simulink model "MicrogridControl"  (R2025b)
settings: Solver=VariableStepAuto  StartTime=0.0  StopTime=8  FixedStep=Ts  RelTol=1e-3
PreLoadFcn:
  | NormalOperation;
  | MicrogridControlParam;
undefined symbols (not defined in the file): base, bessModeInitial, bessSystem, bessVoltage, breakerStatus, DiscIntNeverNeededParam, ee_sli_rtmsupport, event, gcbh, generator, gflInverter, gfmInverter, Inertia, lineInductance, lineResistance, machine, plannedIsland, pmsm, powerLimit, powerQuality, PV, PVInverter, ref, resync, solar, solarInsolationChange, systemFrequency, Ts, windController, windSystem, windTurbine
libraries: nesl_utility x234, ee_lib x174, fl_lib x143, eeGeneralControl x137, simulink x78, eeTransforms x47, slpidlib x23, nesl_utility_internal x12, eePwmGenerator x9, eeSinusoidalMeasurementV2 x9, custom_lib x7, batteryecm_lib x6
(part 4 of 25)

== system MicrogridControl/Wind Farm ==
  Constant : Constant  Value=10
  Constant1 : Constant  Value=0
  Constant2 : Constant  Value=12
  Transformer : Subsystem  Variant=on  VariantControlMode=label  LabelModeActiveChoice=Detailed  mask{fidelity=Detailed}
      mask prompts: fidelity "Modeling Option"
      mask TypeOptions fidelity: Detailed | Simplified
      mask Callback fidelity:
      | choice = get_param(gcb,'fidelity');
      | switch choice
      |     case 'Detailed'
      |         set_param(gcb, 'LabelModeActiveChoice', 'Detailed');
      |     case 'Simplified'
      |          set_param(gcb, 'LabelModeActiveChoice', 'Simplified');
      |     otherwise
      |         disp('Choose proper variant');
      | end
  Transformer1 : Subsystem  Variant=on  VariantControlMode=label  LabelModeActiveChoice=Detailed  mask{fidelity=Detailed}
      mask prompts: fidelity "Modeling Option"
      mask TypeOptions fidelity: Detailed | Simplified
      mask Callback fidelity:
      | choice = get_param(gcb,'fidelity');
      | switch choice
      |     case 'Detailed'
      |         set_param(gcb, 'LabelModeActiveChoice', 'Detailed');
      |     case 'Simplified'
      |          set_param(gcb, 'LabelModeActiveChoice', 'Simplified');
      |     otherwise
      |         disp('Choose proper variant');
      | end
  Wind Plant Integrated : Subsystem  Variant=on  VariantControlMode=label  LabelModeActiveChoice=Detailed  mask(Wind){fidelity=Detailed, plantRating=windSystem.plantRating, Vac=windSystem.Vac, frequency=windSystem.frequency, iMaxPU=windSystem.iMaxPU, efficiency=windSystem.converterEfficiency, baseVoltageDC=windSystem.Vdc, airDensity=windTurbine.airDensity, turbineRadius=windTurbine.turbineRadius, pitch=windTurbine.pitch, TSR=windTurbine.TSR, cp=windTurbine.cp, wt=windTurbine.wThreshold, rt=windTurbine.wThreshold, p=pmsm.polePairs, psim=pmsm.fluxLinkage, Rs=pmsm.Rs, Ld=pmsm.Ld, Lq=pmsm.Lq, capacitance=windSystem.capacitance, filterInductance=windSystem.filterInductance, filterResistance=windSystem.filterResistance, converterFidelity=Average, fSw=20}
      mask prompts: fidelity "Modeling Option"; plantRating "Wind Farm Rating (kW)"; Vac "Rated AC side voltage (phase-phase RMS) (V)"; frequency "Rated electrical frequency at AC side (Hz)"; iMaxPU "Maximum converter current (pu)"; efficiency "Converter Efficiency (%)"; baseVoltageDC "Voltage on DC side (V)"; airDensity "Air density (kg/m^3)"; turbineRadius "Turbine radius (m)"; pitch "Pitch angle vector (deg)"; TSR "Tip speed ratio"; cp "Power coefficient table, Cp(beta,TSR)"; wt "Wind velocity threshold (m/s)"; rt "Rotational velocity threshold (rad/s)"; p "Number of pole pairs"; psim "PMSM flux linkage (Wb)"; Rs "Stator resistance (Ohm)"; Ld "Stator d-axis inductance (H)"; Lq "Stator q-axis inductance (H)"; capacitance "DC bus capacitance (F)"; filterInductance "Filter inductance (H)"; filterResistance "Filter series resistance (Ohm)"; converterFidelity "Converter Fidelity"; fSw "Switching Frequency (kHz)"
      mask help: This block models a detailed Type -4 ind farm with the MPPT Controller. The wind farm comprises a permanent magnnet synhronous machine connected to the main grid via back-to-back converters. Select simplified mode for faster simulation using fixed efficiency and rated power.
      settings: CopyFcn=set_param(gcbh,'LinkStatus','none');
      mask Help: web('WindFarm.html')
      mask TypeOptions fidelity: Detailed | Simplified
      mask Callback fidelity:
      | detailedTabs = {'windDetailed','controllerDetailed','converter'};
      |     simplifiedTabs = {'windSimplified'};
      |     component.mask.fidelitySelection(detailedTabs,simplifiedTabs);
      mask TypeOptions airDensity: Detailed/Wind System/airDensity
      mask TypeOptions turbineRadius: Detailed/Wind System/turbineRadius
      mask TypeOptions pitch: Detailed/Wind System/pitch
      mask TypeOptions TSR: Detailed/Wind System/TSR
      mask TypeOptions cp: Detailed/Wind System/cp
      mask TypeOptions wt: Detailed/Wind System/wt
      mask TypeOptions rt: Detailed/Wind System/rt
      mask TypeOptions p: Detailed/Wind System/p
      mask TypeOptions psim: Detailed/Wind System/psim
      mask TypeOptions Rs: Detailed/Wind System/Rs
      mask TypeOptions Ld: Detailed/Wind System/Ld
      mask TypeOptions Lq: Detailed/Wind System/Lq
      mask TypeOptions converterFidelity: Detailed/Wind Turbine and Converters/Wind Plant/converterFidelity
      mask Callback converterFidelity:
      | converterFidelity = get_param(gcb,'converterFidelity');
      | blockPath = [gcb,'/','Detailed','/','Wind Turbine and Converters','/','Wind Plant','/','Back-to-Back Converters'];
      | % if strcmp(converterFidelity,'Average')
      | %     blockPath = [gcb,'/','Detailed','/','Wind Turbine and Converters','/','Wind Plant','/','Back-to-Back Converters'];
      | % else
      | %     blockPath = [gcb,'/','Detailed','/','Wind Turbine and Converters','/','Wind Plant','/','Back-to-Back Converters'];
      | % end
      | component.mask.converterFidelity(blockPath)
      mask TypeOptions fSw: Detailed/Wind Turbine and Converters/Wind Plant/fSw
      mask DialogControl generalDetailed Prompt: General
      mask DialogControl windDetailed Prompt: Wind Turbine
      mask DialogControl configureWindTurbine Prompt: Edit wind turbine parameters
      mask DialogControl configureWindTurbine Callback:
      | blockPath = [gcb,'/','Detailed','/','Wind Turbine and Converters','/','Wind Plant','/','Wind Turbine'];
      |     component.mask.openBlock(blockPath);
      mask DialogControl Container10 Prompt: PMSM
      mask DialogControl configurePMSM Prompt: Edit PMSM parameters
      mask DialogControl configurePMSM Callback:
      | blockPath = [gcb,'/','Detailed','/','Wind Turbine and Converters','/','Wind Plant','/','PMSG'];
      |  component.mask.openBlock(blockPath);
      mask DialogControl controllerDetailed Prompt: Controller
      mask DialogControl configureWindController Prompt: Edit Wind Controller
      mask DialogControl configureWindController Callback:
      | blockPath = [gcb,'/','Detailed','/','Wind Turbine and Converters','/','Wind Controller'];
      |     component.mask.openBlock(blockPath);
      mask DialogControl windSimplified Prompt: Wind Turbine
      mask DialogControl editWindFarm Prompt: Edit wind farm
      mask DialogControl editWindFarm Callback:
      | blockPath = [gcb,'/','Simplified','/','Wind farm'];
      | component.mask.openBlock(blockPath);
      mask DialogControl converter Prompt: Converter
      mask DialogControl editMSConverter Prompt: Edit machine side converter parameters
      mask DialogControl editMSConverter Callback:
      | blockFidelity = get_param(gcb,'fidelity');
      | converterFidelity = get_param(gcb,'converterFidelity');
      | if strcmp(converterFidelity,'Average')
      |     blockPath = [gcb,'/',blockFidelity,'/','Wind Turbine and Converters','/','Wind Plant','/','Back-to-Back Converters','/',converterFidelity,'/','Machine Side Converter'];
      | else
      |     blockPath = [gcb,'/',blockFidelity,'/','Wind Turbine and Converters','/','Wind Plant','/','Back-to-Back Converters','/',converterFidelity,'/','Machine Side Converter','/','Converter'];
      | end
      | component.mask.openBlock(blockPath);
      mask DialogControl editGSConverter Prompt: Edit grid side converter parameters
      mask DialogControl editGSConverter Callback:
      | blockFidelity = get_param(gcb,'fidelity');
      | converterFidelity = get_param(gcb,'converterFidelity');
      | if strcmp(converterFidelity,'Average')
      |     blockPath = [gcb,'/',blockFidelity,'/','Wind Turbine and Converters','/','Wind Plant','/','Back-to-Back Converters','/',converterFidelity,'/','Grid Side Converter'];
      | else
      |     blockPath = [gcb,'/',blockFidelity,'/','Wind Turbine and Converters','/','Wind Plant','/','Back-to-Back Converters','/',converterFidelity,'/','Grid Side Converter','/','Converter'];
      | end
      | component.mask.openBlock(blockPath);
      mask Display: image('wind_plant.png');
  Wind Plant Integrated1 : Subsystem  Variant=on  VariantControlMode=label  LabelModeActiveChoice=Detailed  mask(Wind){fidelity=Detailed, plantRating=windSystem.plantRating, Vac=windSystem.Vac, frequency=windSystem.frequency, iMaxPU=windSystem.iMaxPU, efficiency=windSystem.converterEfficiency, baseVoltageDC=windSystem.Vdc, airDensity=windTurbine.airDensity, turbineRadius=windTurbine.turbineRadius, pitch=windTurbine.pitch, TSR=windTurbine.TSR, cp=windTurbine.cp, wt=windTurbine.wThreshold, rt=windTurbine.wThreshold, p=pmsm.polePairs, psim=pmsm.fluxLinkage, Rs=pmsm.Rs, Ld=pmsm.Ld, Lq=pmsm.Lq, capacitance=windSystem.capacitance, filterInductance=windSystem.filterInductance, filterResistance=windSystem.filterResistance, converterFidelity=Average, fSw=20}
      mask prompts: fidelity "Modeling Option"; plantRating "Wind Farm Rating (kW)"; Vac "Rated AC side voltage (phase-phase RMS) (V)"; frequency "Rated electrical frequency at AC side (Hz)"; iMaxPU "Maximum converter current (pu)"; efficiency "Converter Efficiency (%)"; baseVoltageDC "Voltage on DC side (V)"; airDensity "Air density (kg/m^3)"; turbineRadius "Turbine radius (m)"; pitch "Pitch angle vector (deg)"; TSR "Tip speed ratio"; cp "Power coefficient table, Cp(beta,TSR)"; wt "Wind velocity threshold (m/s)"; rt "Rotational velocity threshold (rad/s)"; p "Number of pole pairs"; psim "PMSM flux linkage (Wb)"; Rs "Stator resistance (Ohm)"; Ld "Stator d-axis inductance (H)"; Lq "Stator q-axis inductance (H)"; capacitance "DC bus capacitance (F)"; filterInductance "Filter inductance (H)"; filterResistance "Filter series resistance (Ohm)"; converterFidelity "Converter Fidelity"; fSw "Switching Frequency (kHz)"
      mask help: This block models a detailed Type -4 ind farm with the MPPT Controller. The wind farm comprises a permanent magnnet synhronous machine connected to the main grid via back-to-back converters. Select simplified mode for faster simulation using fixed efficiency and rated power.
      settings: CopyFcn=set_param(gcbh,'LinkStatus','none');
      mask Help: web('WindFarm.html')
      mask TypeOptions fidelity: Detailed | Simplified
      mask Callback fidelity:
      | detailedTabs = {'windDetailed','controllerDetailed','converter'};
      |     simplifiedTabs = {'windSimplified'};
      |     component.mask.fidelitySelection(detailedTabs,simplifiedTabs);
      mask TypeOptions airDensity: Detailed/Wind System/airDensity
      mask TypeOptions turbineRadius: Detailed/Wind System/turbineRadius
      mask TypeOptions pitch: Detailed/Wind System/pitch
      mask TypeOptions TSR: Detailed/Wind System/TSR
      mask TypeOptions cp: Detailed/Wind System/cp
      mask TypeOptions wt: Detailed/Wind System/wt
      mask TypeOptions rt: Detailed/Wind System/rt
      mask TypeOptions p: Detailed/Wind System/p
      mask TypeOptions psim: Detailed/Wind System/psim
      mask TypeOptions Rs: Detailed/Wind System/Rs
      mask TypeOptions Ld: Detailed/Wind System/Ld
      mask TypeOptions Lq: Detailed/Wind System/Lq
      mask TypeOptions converterFidelity: Detailed/Wind Turbine and Converters/Wind Plant/converterFidelity
      mask Callback converterFidelity:
      | converterFidelity = get_param(gcb,'converterFidelity');
      | blockPath = [gcb,'/','Detailed','/','Wind Turbine and Converters','/','Wind Plant','/','Back-to-Back Converters'];
      | % if strcmp(converterFidelity,'Average')
      | %     blockPath = [gcb,'/','Detailed','/','Wind Turbine and Converters','/','Wind Plant','/','Back-to-Back Converters'];
      | % else
      | %     blockPath = [gcb,'/','Detailed','/','Wind Turbine and Converters','/','Wind Plant','/','Back-to-Back Converters'];
      | % end
      | component.mask.converterFidelity(blockPath)
      mask TypeOptions fSw: Detailed/Wind Turbine and Converters/Wind Plant/fSw
      mask DialogControl generalDetailed Prompt: General
      mask DialogControl windDetailed Prompt: Wind Turbine
      mask DialogControl configureWindTurbine Prompt: Edit wind turbine parameters
      mask DialogControl configureWindTurbine Callback:
      | blockPath = [gcb,'/','Detailed','/','Wind Turbine and Converters','/','Wind Plant','/','Wind Turbine'];
      |     component.mask.openBlock(blockPath);
      mask DialogControl Container10 Prompt: PMSM
      mask DialogControl configurePMSM Prompt: Edit PMSM parameters
      mask DialogControl configurePMSM Callback:
      | blockPath = [gcb,'/','Detailed','/','Wind Turbine and Converters','/','Wind Plant','/','PMSG'];
      |  component.mask.openBlock(blockPath);
      mask DialogControl controllerDetailed Prompt: Controller
      mask DialogControl configureWindController Prompt: Edit Wind Controller
      mask DialogControl configureWindController Callback:
      | blockPath = [gcb,'/','Detailed','/','Wind Turbine and Converters','/','Wind Controller'];
      |     component.mask.openBlock(blockPath);
      mask DialogControl windSimplified Prompt: Wind Turbine
      mask DialogControl editWindFarm Prompt: Edit wind farm
      mask DialogControl editWindFarm Callback:
      | blockPath = [gcb,'/','Simplified','/','Wind farm'];
      | component.mask.openBlock(blockPath);
      mask DialogControl converter Prompt: Converter
      mask DialogControl editMSConverter Prompt: Edit machine side converter parameters
      mask DialogControl editMSConverter Callback:
      | blockFidelity = get_param(gcb,'fidelity');
      | converterFidelity = get_param(gcb,'converterFidelity');
      | if strcmp(converterFidelity,'Average')
      |     blockPath = [gcb,'/',blockFidelity,'/','Wind Turbine and Converters','/','Wind Plant','/','Back-to-Back Converters','/',converterFidelity,'/','Machine Side Converter'];
      | else
      |     blockPath = [gcb,'/',blockFidelity,'/','Wind Turbine and Converters','/','Wind Plant','/','Back-to-Back Converters','/',converterFidelity,'/','Machine Side Converter','/','Converter'];
      | end
      | component.mask.openBlock(blockPath);
      mask DialogControl editGSConverter Prompt: Edit grid side converter parameters
      mask DialogControl editGSConverter Callback:
      | blockFidelity = get_param(gcb,'fidelity');
      | converterFidelity = get_param(gcb,'converterFidelity');
      | if strcmp(converterFidelity,'Average')
      |     blockPath = [gcb,'/',blockFidelity,'/','Wind Turbine and Converters','/','Wind Plant','/','Back-to-Back Converters','/',converterFidelity,'/','Grid Side Converter'];
      | else
      |     blockPath = [gcb,'/',blockFidelity,'/','Wind Turbine and Converters','/','Wind Plant','/','Back-to-Back Converters','/',converterFidelity,'/','Grid Side Converter','/','Converter'];
      | end
      | component.mask.openBlock(blockPath);
      mask Display: image('wind_plant.png');
  ~ : PMIOPort  Side=Left
  wires:
  Constant1/1 -> Wind Plant Integrated1/2(QRef), Wind Plant Integrated/2(QRef)
  Constant/1 -> Wind Plant Integrated1/1(LVRT), Wind Plant Integrated/1(LVRT)
  Constant2/1 -> Wind Plant Integrated1/3(WindSpeed), Wind Plant Integrated/3(WindSpeed)
  connections:
  ~/RConn1 -- Transformer1/RConn1 -- Transformer/RConn1
  Wind Plant Integrated/RConn1 -- Transformer/LConn1
  Wind Plant Integrated1/RConn1 -- Transformer1/LConn1

== system MicrogridControl/BESS/BESS Integrated ==
  VRef : Inport
  FRef : Inport  Port=2
  PRef : Inport  Port=3
  QRef : Inport  Port=4
  Mode : Inport  Port=5
  Reset : Inport  Port=6
  Detailed : Subsystem  VariantControl=Detailed
  Simplified : Subsystem  Variant=on  VariantControlMode=label  VariantControl=Simplified  LabelModeActiveChoice=Grid Forming
  ~ : PMIOPort  Side=Right
  Meas : Outport

== system MicrogridControl/BESS/BESS Integrated1 ==
  VRef : Inport
  FRef : Inport  Port=2
  PRef : Inport  Port=3
  QRef : Inport  Port=4
  Mode : Inport  Port=5
  Reset : Inport  Port=6
  Detailed : Subsystem  VariantControl=Detailed
  Simplified : Subsystem  Variant=on  VariantControlMode=label  VariantControl=Simplified  LabelModeActiveChoice=Grid Forming
  ~ : PMIOPort  Side=Right
  Meas : Outport

== system MicrogridControl/BESS/BESS Integrated3 ==
  VRef : Inport
  FRef : Inport  Port=2
  PRef : Inport  Port=3
  QRef : Inport  Port=4
  Mode : Inport  Port=5
  Reset : Inport  Port=6
  Detailed : Subsystem  VariantControl=Detailed
  Simplified : Subsystem  Variant=on  VariantControlMode=label  VariantControl=Simplified  LabelModeActiveChoice=Grid Forming
  ~ : PMIOPort  Side=Right
  Meas : Outport

== system MicrogridControl/BESS/Transformer ==
  Detailed : Subsystem  VariantControl=Detailed
  Simplified : Subsystem  VariantControl=Simplified  mask{windingRatio=690/6600}
      mask prompts: windingRatio "Winding ratio"
      mask DialogControl Container4 Prompt: General
  In : PMIOPort  Side=Left
  Out : PMIOPort  Port=2  Side=Right

== system MicrogridControl/BESS/Transformer1 ==
  Detailed : Subsystem  VariantControl=Detailed
  Simplified : Subsystem  VariantControl=Simplified  mask{windingRatio=690/6600}
      mask prompts: windingRatio "Winding ratio"
      mask DialogControl Container4 Prompt: General
  In : PMIOPort  Side=Left
  Out : PMIOPort  Port=2  Side=Right

== system MicrogridControl/BESS/Transformer3 ==
  Detailed : Subsystem  VariantControl=Detailed
  Simplified : Subsystem  VariantControl=Simplified  mask{windingRatio=690/6600}
      mask prompts: windingRatio "Winding ratio"
      mask DialogControl Container4 Prompt: General
  In : PMIOPort  Side=Left
  Out : PMIOPort  Port=2  Side=Right

== system MicrogridControl/Domestic Load/Circuit Breaker ==
  BRK : Inport
  Data Type Conversion : DataTypeConversion  OutDataTypeStr=double  SaturateOnIntegerOverflow=off  RndMeth=Floor
  Open Resistance : Gain  Gain=5e6
  Phase Splitter : ee_lib/Connectors & References/Phase Splitter
  Phase Splitter1 : ee_lib/Connectors & References/Phase Splitter
  Simulink-PS Converter : nesl_utility/Simulink-PS Converter  PhysicalDomain=network_engine_domain  SubClassName=ps_input  LeftPortType=input  RightPortType=output  PseudoPeriodic=off  Frequencies=[]  NoiseDistribution=none  NoiseParameters=[]  Unit=1  AffineConversion=off  FilteringAndDerivatives=provide  SimscapeFilterOrder=1  InputFilterTimeConstant=0.001  UdotUserProvided=0
  Variable Resistor : fl_lib/Electrical/Electrical Elements/Variable Resistor  Rmin=1e-3 Ohm  thermalEnable=false  thermal_mass=1 J/K  i_specify=on  i_priority=None  i=0 A  i_nominal_specify=off  i_nominal_value=1  i_nominal_unit=A  v_specify=off  v_priority=None  v=0 V  v_nominal_specify=off  v_nominal_value=1  v_nominal_unit=V  T_specify=off  T_priority=None  T=300 K  T_nominal_specify=off  T_nominal_value=1  T_nominal_unit=K
  Variable Resistor1 : fl_lib/Electrical/Electrical Elements/Variable Resistor  Rmin=1e-3 Ohm  thermalEnable=false  thermal_mass=1 J/K  i_specify=on  i_priority=None  i=0 A  i_nominal_specify=off  i_nominal_value=1  i_nominal_unit=A  v_specify=off  v_priority=None  v=0 V  v_nominal_specify=off  v_nominal_value=1  v_nominal_unit=V  T_specify=off  T_priority=None  T=300 K  T_nominal_specify=off  T_nominal_value=1  T_nominal_unit=K
  Variable Resistor2 : fl_lib/Electrical/Electrical Elements/Variable Resistor  Rmin=1e-3 Ohm  thermalEnable=false  thermal_mass=1 J/K  i_specify=on  i_priority=None  i=0 A  i_nominal_specify=off  i_nominal_value=1  i_nominal_unit=A  v_specify=off  v_priority=None  v=0 V  v_nominal_specify=off  v_nominal_value=1  v_nominal_unit=V  T_specify=off  T_priority=None  T=300 K  T_nominal_specify=off  T_nominal_value=1  T_nominal_unit=K
  In : PMIOPort  Side=Left
  ~ : PMIOPort  Port=2  Side=Right
  wires:
  Data Type Conversion/1 -> Open Resistance/1
  BRK/1 -> Data Type Conversion/1
  Open Resistance/1 -> Simulink-PS Converter/1
  connections:
  Phase Splitter1/RConn2 -- Variable Resistor1/RConn1
  Variable Resistor1/LConn2 -- Phase Splitter/RConn2
  Phase Splitter1/RConn3 -- Variable Resistor2/RConn1
  Phase Splitter/RConn1 -- Variable Resistor/LConn2
  Variable Resistor2/LConn2 -- Phase Splitter/RConn3
  Phase Splitter1/RConn1 -- Variable Resistor/RConn1
  Phase Splitter1/LConn1 -- ~/RConn1
  Variable Resistor/LConn1 -- Simulink-PS Converter/RConn1 -- Variable Resistor2/LConn1 -- Variable Resistor1/LConn1
  Phase Splitter/LConn1 -- In/RConn1

== system MicrogridControl/Generator/Generator Integrated ==
  PRef : Inport
  Detailed : Subsystem  VariantControl=Detailed
  Simplified : Subsystem  VariantControl=Simplified
  ~ : PMIOPort  Side=Right
  Meas : Outport

== system MicrogridControl/Generator/Transformer ==
  Detailed : Subsystem  VariantControl=Detailed
  Simplified : Subsystem  VariantControl=Simplified  mask{windingRatio=690/6600}
      mask prompts: windingRatio "Winding ratio"
      mask DialogControl Container4 Prompt: General
  In : PMIOPort  Side=Left
  Out : PMIOPort  Port=2  Side=Right

== system MicrogridControl/Microgrid Controller/Breaker Control ==
  Bus Element In : Inport  PortName=BrKControl  Element=PCC
  CtrlRm BRK : Inport  Port=2
  Cast To Double1 : DataTypeConversion  OutDataTypeStr=double  SaturateOnIntegerOverflow=off  RndMeth=Floor
  Delay : Delay  DelayLength=1  InitialCondition=breakerStatus.PCCInitial
  Switch : Switch  Criteria=u2 > Threshold  SaturateOnIntegerOverflow=off  InputSameDT=off
  BrK Ctrl : Outport
  wires:
  Delay/1 -> Cast To Double1/1
  Bus Element In/1 -> Delay/1
  CtrlRm BRK/1 -> Switch/1, Switch/2
  Cast To Double1/1 -> Switch/3  "BRK Status"
  Switch/1 -> BrK Ctrl/1  "BRK Status"

== system MicrogridControl/Microgrid Controller/Microgrid Control Functions ==
  BusElementIn3 : Inport  PortName=mPLL  Element=islandVoltage
  BusElementIn4 : Inport  PortName=mPLL  Element=islandFrequency
  BusElementIn6 : Inport  PortName=mPLL  Element=gridFrequency
  BusElementIn : Inport  PortName=mPLL  Element=gridAngle
  BusElementIn1 : Inport  PortName=mPLL  Element=gridVoltage
  BusElementIn2 : Inport  PortName=mPLL  Element=islandAngle
  BESS Reactive Power : Inport  Port=2
  PCC Active Power : Inport  Port=3
  PCC Reactive Power : Inport  Port=4
  Bus Element In1 : Inport  Port=5  PortName=Status  Element=plannedIslandingEnable
  Bus Element In2 : Inport  Port=5  PortName=Status  Element=blackStartEnable
  Bus Element In4 : Inport  Port=5  PortName=Status  Element=resyncEnable
  Bus Element In3 : Inport  Port=5  PortName=Status  Element=resync
  Black Start : Subsystem  mask(BlackStart){referenceFrequency=blackStartFrequency, controllerBlackStart=blackStartTime, voltageLevel1=level1, voltageLevel2=level2, voltageLevel3=level3, delayLevel1=delay1, delayLevel2=delay2, delayLevel3=delay3}
      mask prompts: referenceFrequency "Reference Frequency"; controllerBlackStart "Black Start Time"; voltageLevel1 "Level1"; voltageLevel2 "Level2"; voltageLevel3 "Level3"; delayLevel1 "Delay1"; delayLevel2 "Delay2"; delayLevel3 "Delay3"
      mask help: This block implements the black start logic in the microgrid
      settings: CopyFcn=set_param(gcbh,'LinkStatus','none')
      mask Help: web('BlackStart.html')
      mask DialogControl Container4 Prompt: General
      mask DialogControl Container5 Prompt: Voltage Levels
      mask DialogControl Container6 Prompt: Time Delay
  Latency_Blackstart : Delay  DelayLength=1  SampleTime=Ts
  Latency_PlannedIsland : Delay  DelayLength=1  SampleTime=Ts
  Latency_Resync : Delay  DelayLength=1  SampleTime=Ts
  PlannedIslanding1 : Subsystem  mask(PlannedIslanding){KpPPlannedIsland=kpActive, KiPPlannedIsland=kiActive, ZeroActivePowerThreshold=activeThreshold, KpQPlannedIsland=kpReactive, KiQPlannedIsland=kiReactive, ZeroReactivePowerThreshold=reactiveThreshold}
      mask prompts: KpPPlannedIsland "Proportional Gain"; KiPPlannedIsland "Integral Gain"; ZeroActivePowerThreshold "Threshold"; KpQPlannedIsland "Proportional Gain"; KiQPlannedIsland "Integral Gain"; ZeroReactivePowerThreshold "Threshold"
      mask help: This block enables the microgrid to island from the grid in a planned manner by reducing the active and reactive power from the grid
      settings: CopyFcn=set_param(gcbh,'LinkStatus','none');
      mask Help: web('PlannedIslanding.html')
      mask DialogControl Container4 Prompt: Active Power
      mask DialogControl Container5 Prompt: Reactive Power
  Resynchronization : Subsystem  mask(Resynchronization){GridFrequency=gridFrequency, KpVolResynch=kpVoltage, KiVolResynch=kiVoltage, VoltageThreshold=voltageThreshold, kDroop=voltageDroop, KpFreResynch=kpFrequency, KiFreResynch=kpFrequency, FrequencyThreshold=frequencyThreshold, KpAngResynch=kpAngle, KiAngResynch=kiAngle, AngleThreshold=angleThreshold}
      mask prompts: GridFrequency "Grid Frequency"; KpVolResynch "Proportional Gain"; KiVolResynch "Integral Gain"; kDroop "Voltage Droop"; KpFreResynch "Proportional Gain"; KiFreResynch "Integral Gain"; KpAngResynch "Proportional Gain"; KiAngResynch "Integral Gain"
      mask help: This block enables the microgrid to reconnect with the grid if the voltage, frequency and angle of the islanded microgrid matches to the grid with certain threshold
      settings: CopyFcn=set_param(gcbh,'LinkStatus','none');
      mask Help: web('Resynchronization.html')
      mask DialogControl Container4 Prompt: General
      mask DialogControl Container6 Prompt: Voltage
      mask DialogControl Container5 Prompt: Frequency
      mask DialogControl Container7 Prompt: Angle
  Resync : Outport
  PlannedIslanding : Outport  Port=2
  BlackStart : Outport  Port=3
  Resync Status : Outport  Port=4
  PlannedIsland Status : Outport  Port=5
  BlackStart Status : Outport  Port=6
  wires:
  Bus Element In4/1 -> Resynchronization/1(Enable)
  BESS Reactive Power/1 -> Resynchronization/2(BESS Reactive Power)
  Bus Element In3/1 -> Resynchronization/3(Resynch BreakerEnable)
  BusElementIn1/1 -> Resynchronization/4(Grid Voltage)
  BusElementIn6/1 -> Resynchronization/5(Grid Frequency)
  BusElementIn/1 -> Resynchronization/6(Grid Angle)
  BusElementIn3/1 -> Black Start/2(Voltage), Resynchronization/7(Island Voltage)
  BusElementIn4/1 -> Resynchronization/8(Island Frequency)
  BusElementIn2/1 -> Resynchronization/9(Island Angle)
  Resynchronization/2(Resync) -> Resync/1  "Resync"
  Resynchronization/1(Status) -> Latency_Resync/1
  Latency_Resync/1 -> Resync Status/1
  Bus Element In1/1 -> PlannedIslanding1/1(Enable)
  PCC Active Power/1 -> PlannedIslanding1/2(P)
  PCC Reactive Power/1 -> PlannedIslanding1/3(Q)
  PlannedIslanding1/1(Status) -> Latency_PlannedIsland/1
  Latency_PlannedIsland/1 -> PlannedIsland Status/1
  PlannedIslanding1/2(PlannedIslanding) -> PlannedIslanding/1  "PlannedIslanding"
  Bus Element In2/1 -> Black Start/1(Enable)
  Black Start/1(BlackStart) -> Latency_Blackstart/1  "BlackStart"
  Latency_Blackstart/1 -> BlackStart/1
  Black Start/2(Status) -> BlackStart Status/1

== system MicrogridControl/Microgrid Controller/Microgrid Supervisory Control ==
  Resync Status : Inport
  PlannedIslanding Status : Inport  Port=2
  BlackStart Status : Inport  Port=3
  Resync Enable : Inport  Port=4
  PlannedIslandEnable : Inport  Port=5
  UnplannedIslandingEnable : Inport  Port=6
  BlackStart Enable : Inport  Port=7
  Blackout Status : Inport  Port=8
  BusElementIn : Inport  Port=9  PortName=mPLL  Element=islandVoltage
  BusElementIn1 : Inport  Port=9  PortName=mPLL  Element=islandFrequency
  BreakerStatus : Inport  Port=10
  Bus Assignment : BusAssignment  AssignedSignals=mode
  Bus Creator : BusCreator  Inputs=3
  Bus Creator1 : BusCreator  Inputs=2
  Bus Creator2 : BusCreator  Inputs=3
  Bus Creator3 : BusCreator  Inputs=3
  Constant : Constant  Value=resyncDelay
  Constant1 : Constant  Value=plannedIslandingDelay
  Delay : Delay  DelayLength=1  InitialCondition=breakerStatus.PCCInitial  SampleTime=Ts
  Scope1 : Scope  NumInputPorts=2
      settings: ActiveDisplayYMinimum=-0.14534871395899834  ActiveDisplayYMaximum=1.3081384256309854  DataLoggingVariableName=ScopeData17
  Transition and Dispatch Control : Stateflow chart  TreatAsAtomicUnit=on  mask(Microgrid Transition and Dispatch Control){upperVoltageLimit=upperVoltagelimit, lowerVoltageLimit=lowerVoltageLimit, upperFrequencyLimit=upperFrequencyLimit, lowerFrequencyLimit=lowerFrequencyLimit}
      mask prompts: upperVoltageLimit "Max Voltage in pu"; lowerVoltageLimit "Min Voltage in pu"; upperFrequencyLimit "Max Frequency in Hz"; lowerFrequencyLimit "Min Frequency in Hz"
      mask help: This subsystem implements the transitions and the corresponding dispatch functions in the microgrid
  BrKControl : Outport
  Status : Outport  Port=2
  wires:
  PlannedIslanding Status/1 -> Bus Creator2/2  "status"
  PlannedIslandEnable/1 -> Bus Creator2/1  "enable"
  UnplannedIslandingEnable/1 -> Transition and Dispatch Control/2(UnplannedIslandingEnable)
  Bus Creator1/1 -> Transition and Dispatch Control/3(Island)  "Island"
  BusElementIn1/1 -> Scope1/2, Bus Creator1/2  "frequency"
  BusElementIn/1 -> Scope1/1, Bus Creator1/1  "voltage"
  Bus Creator/1 -> Transition and Dispatch Control/1(Resync)  "Resync"
  Constant/1 -> Bus Creator/3  "delay"
  Resync Status/1 -> Bus Creator/2  "status"
  Resync Enable/1 -> Bus Creator/1  "enable"
  Transition and Dispatch Control/1(BrKControl) -> BrKControl/1  "BrKControl"
  BreakerStatus/1 -> Delay/1
  Transition and Dispatch Control/2(Status) -> Bus Assignment/1
  Bus Assignment/1 -> Status/1  "Status"
  Delay/1 -> Transition and Dispatch Control/4(BreakerStatus)
  Constant1/1 -> Bus Creator2/3  "delay"
  BlackStart Status/1 -> Bus Creator3/2  "status"
  Blackout Status/1 -> Bus Creator3/3  "blackout"
  BlackStart Enable/1 -> Bus Creator3/1  "enable"
  Bus Creator3/1 -> Transition and Dispatch Control/6(BlackStart)  "BlackStart"
  Bus Creator2/1 -> Transition and Dispatch Control/5(PlannedIslanding)  "PlannedIslanding"
  Transition and Dispatch Control/3(Transition_and_Dispatch_ControlMode) -> Bus Assignment/2

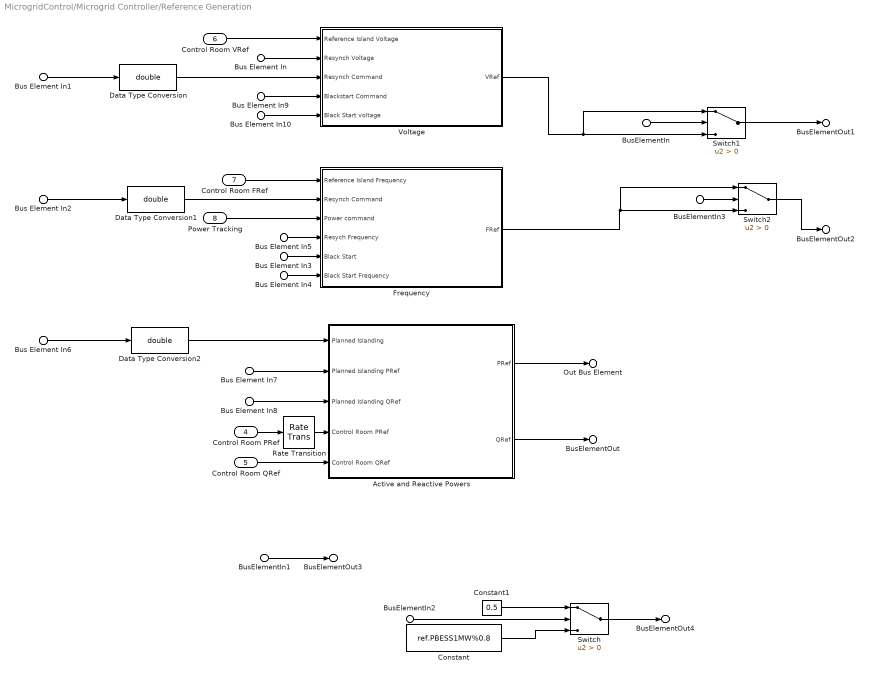
== system MicrogridControl/Microgrid Controller/Reference Generation ==
  Bus Element In : Inport  PortName=Resync  Element=synchVoltagedpr
  Bus Element In5 : Inport  PortName=Resync  Element=synchFrequency
  Bus Element In7 : Inport  Port=2  PortName=Planned Islanding  Element=activePower
  Bus Element In8 : Inport  Port=2  PortName=Planned Islanding  Element=reactivePower
  Bus Element In3 : Inport  Port=3  PortName=BlackStart  Element=enableCommand
  Bus Element In9 : Inport  Port=3  PortName=BlackStart  Element=enableCommand
  Bus Element In4 : Inport  Port=3  PortName=BlackStart  Element=Fref
  Bus Element In10 : Inport  Port=3  PortName=BlackStart  Element=Vref
  Control Room PRef : Inport  Port=4
  Control Room QRef : Inport  Port=5
  Control Room VRef : Inport  Port=6
  Control Room FRef : Inport  Port=7
  Power Tracking : Inport  Port=8
  Bus Element In6 : Inport  Port=9  PortName=Status  Element=plannedIslandingEnable
  Bus Element In1 : Inport  Port=9  PortName=Status  Element=resyncEnable
  Bus Element In2 : Inport  Port=9  PortName=Status  Element=resyncEnable
  BusElementIn1 : Inport  Port=9  PortName=Status  Element=bessMode
  BusElementIn2 : Inport  Port=9  PortName=Status  Element=resync
  BusElementIn : Inport  Port=9  PortName=Status  Element=resync
  BusElementIn3 : Inport  Port=9  PortName=Status  Element=resync
  Active and Reactive Powers : Subsystem
  Constant : Constant  Value=ref.PBESS1MW%0.8
  Constant1 : Constant  Value=0.5
  Data Type Conversion : DataTypeConversion  OutDataTypeStr=double  SaturateOnIntegerOverflow=off  RndMeth=Floor
  Data Type Conversion1 : DataTypeConversion  OutDataTypeStr=double  SaturateOnIntegerOverflow=off  RndMeth=Floor
  Data Type Conversion2 : DataTypeConversion  OutDataTypeStr=double  SaturateOnIntegerOverflow=off  RndMeth=Floor
  Frequency : Subsystem
  Rate Transition : RateTransition  OutPortSampleTime=1e-3
  Switch : Switch  Criteria=u2 > Threshold  SaturateOnIntegerOverflow=off  InputSameDT=off
  Switch1 : Switch  Criteria=u2 > Threshold  SaturateOnIntegerOverflow=off  InputSameDT=off
  Switch2 : Switch  Criteria=u2 > Threshold  SaturateOnIntegerOverflow=off  InputSameDT=off
  Voltage : Subsystem
  Out Bus Element : Outport  PortName=ref  Element=activePower
  BusElementOut : Outport  PortName=ref  Element=reactivePower
  BusElementOut1 : Outport  PortName=ref  Element=voltage
  BusElementOut2 : Outport  PortName=ref  Element=frequency
  BusElementOut3 : Outport  PortName=ref  Element=mode
  BusElementOut4 : Outport  PortName=ref  Element=activePowerBESS1
  wires:
  Control Room FRef/1 -> Frequency/1(Reference Island Frequency)
  Bus Element In7/1 -> Active and Reactive Powers/2(Planned Islanding PRef)
  Control Room PRef/1 -> Rate Transition/1
  Bus Element In9/1 -> Voltage/4(Blackstart Command)
  Bus Element In10/1 -> Voltage/5(Black Start voltage)
  Bus Element In2/1 -> Data Type Conversion1/1
  Data Type Conversion1/1 -> Frequency/2(Resynch Command)
  Bus Element In/1 -> Voltage/2(Resynch Voltage)
  Bus Element In5/1 -> Frequency/4(Resych Frequency)
  Bus Element In8/1 -> Active and Reactive Powers/3(Planned Islanding QRef)
  Rate Transition/1 -> Active and Reactive Powers/4(Control Room PRef)
  Bus Element In3/1 -> Frequency/5(Black Start)
  Control Room QRef/1 -> Active and Reactive Powers/5(Control Room QRef)
  Control Room VRef/1 -> Voltage/1(Reference Island Voltage)
  Data Type Conversion2/1 -> Active and Reactive Powers/1(Planned Islanding)
  Bus Element In4/1 -> Frequency/6(Black Start Frequency)
  Data Type Conversion/1 -> Voltage/3(Resynch Command)
  Bus Element In1/1 -> Data Type Conversion/1
  Power Tracking/1 -> Frequency/3(Power command)
  Bus Element In6/1 -> Data Type Conversion2/1
  Active and Reactive Powers/1(PRef) -> Out Bus Element/1
  Active and Reactive Powers/2(QRef) -> BusElementOut/1
  BusElementIn2/1 -> Switch/2
  BusElementIn1/1 -> BusElementOut3/1
  Constant/1 -> Switch/3
  Switch/1 -> BusElementOut4/1
  Constant1/1 -> Switch/1
  BusElementIn/1 -> Switch1/2
  Voltage/1(VRef) -> Switch1/1, Switch1/3
  BusElementIn3/1 -> Switch2/2
  Switch1/1 -> BusElementOut1/1
  Switch2/1 -> BusElementOut2/1
  Frequency/1(FRef) -> Switch2/1, Switch2/3

== system MicrogridControl/Microgrid Controller/Subsystem1 ==
  Grid Voltage : Inport
  PCC Voltage : Inport  Port=2
  PLL : Subsystem
  PLL start at 0.2 s : Subsystem
  PLL starts at 0.2 s : Subsystem
  PLL1 : Subsystem
  Out Bus Element5 : Outport  PortName=mPLL  Element=islandVoltage
  Out Bus Element3 : Outport  PortName=mPLL  Element=islandFrequency
  Out Bus Element : Outport  PortName=mPLL  Element=gridFrequency
  Out Bus Element1 : Outport  PortName=mPLL  Element=gridAngle
  Out Bus Element2 : Outport  PortName=mPLL  Element=gridVoltage
  Out Bus Element4 : Outport  PortName=mPLL  Element=islandAngle
  wires:
  PLL start at 0.2 s/1(Out1) -> PLL/1(abc)
  PLL starts at 0.2 s/1(abc) -> PLL1/1(abc)
  PLL/3(mag) -> Out Bus Element2/1
  PLL/1(fre) -> Out Bus Element/1
  PLL1/3(mag) -> Out Bus Element5/1
  PLL/2(angle) -> Out Bus Element1/1
  PLL1/1(fre) -> Out Bus Element3/1
  Grid Voltage/1 -> PLL start at 0.2 s/1(PCC measurement)
  PCC Voltage/1 -> PLL starts at 0.2 s/1(PCC measurement)
  PLL1/2(angle) -> Out Bus Element4/1

== system MicrogridControl/Motor Load/Circuit Breaker ==
  BRK : Inport
  Data Type Conversion : DataTypeConversion  OutDataTypeStr=double  SaturateOnIntegerOverflow=off  RndMeth=Floor
  Open Resistance : Gain  Gain=5e6
  Phase Splitter : ee_lib/Connectors & References/Phase Splitter
  Phase Splitter1 : ee_lib/Connectors & References/Phase Splitter
  Simulink-PS Converter : nesl_utility/Simulink-PS Converter  PhysicalDomain=network_engine_domain  SubClassName=ps_input  LeftPortType=input  RightPortType=output  PseudoPeriodic=off  Frequencies=[]  NoiseDistribution=none  NoiseParameters=[]  Unit=1  AffineConversion=off  FilteringAndDerivatives=provide  SimscapeFilterOrder=1  InputFilterTimeConstant=0.001  UdotUserProvided=0
  Variable Resistor : fl_lib/Electrical/Electrical Elements/Variable Resistor  Rmin=1e-3 Ohm  thermalEnable=false  thermal_mass=1 J/K  i_specify=on  i_priority=None  i=0 A  i_nominal_specify=off  i_nominal_value=1  i_nominal_unit=A  v_specify=off  v_priority=None  v=0 V  v_nominal_specify=off  v_nominal_value=1  v_nominal_unit=V  T_specify=off  T_priority=None  T=300 K  T_nominal_specify=off  T_nominal_value=1  T_nominal_unit=K
  Variable Resistor1 : fl_lib/Electrical/Electrical Elements/Variable Resistor  Rmin=1e-3 Ohm  thermalEnable=false  thermal_mass=1 J/K  i_specify=on  i_priority=None  i=0 A  i_nominal_specify=off  i_nominal_value=1  i_nominal_unit=A  v_specify=off  v_priority=None  v=0 V  v_nominal_specify=off  v_nominal_value=1  v_nominal_unit=V  T_specify=off  T_priority=None  T=300 K  T_nominal_specify=off  T_nominal_value=1  T_nominal_unit=K
  Variable Resistor2 : fl_lib/Electrical/Electrical Elements/Variable Resistor  Rmin=1e-3 Ohm  thermalEnable=false  thermal_mass=1 J/K  i_specify=on  i_priority=None  i=0 A  i_nominal_specify=off  i_nominal_value=1  i_nominal_unit=A  v_specify=off  v_priority=None  v=0 V  v_nominal_specify=off  v_nominal_value=1  v_nominal_unit=V  T_specify=off  T_priority=None  T=300 K  T_nominal_specify=off  T_nominal_value=1  T_nominal_unit=K
  In : PMIOPort  Side=Left
  ~ : PMIOPort  Port=2  Side=Right
  wires:
  Data Type Conversion/1 -> Open Resistance/1
  BRK/1 -> Data Type Conversion/1
  Open Resistance/1 -> Simulink-PS Converter/1
  connections:
  Phase Splitter1/RConn2 -- Variable Resistor1/RConn1
  Variable Resistor1/LConn2 -- Phase Splitter/RConn2
  Phase Splitter1/RConn3 -- Variable Resistor2/RConn1
  Phase Splitter/RConn1 -- Variable Resistor/LConn2
  Variable Resistor2/LConn2 -- Phase Splitter/RConn3
  Phase Splitter1/RConn1 -- Variable Resistor/RConn1
  Phase Splitter1/LConn1 -- ~/RConn1
  Variable Resistor/LConn1 -- Simulink-PS Converter/RConn1 -- Variable Resistor2/LConn1 -- Variable Resistor1/LConn1
  Phase Splitter/LConn1 -- In/RConn1

== system MicrogridControl/Motor Load/Motor Loads ==
  Asynchronous Machine Squirrel Cage (fundamental) : ee_lib/Electromechanical/Asynchronous/Induction Machine Squirrel Cage  port_option=ee.enum.threePhasePort.composite  SRated=3e6 V*A  VRated=11000 V  FRated=50 Hz  nPolePairs=1  param_unit=ee.enum.unit.si  squirrel_cage=ee.enum.squirrelcage.Single  zero_sequence=ee.enum.park.zerosequence.exclude  initialization_option=ee.enum.asm.initialization.fluxvariables  Rs=0.016744*10 Ohm  Xls=0.035490*10 Ohm  pu_Rs=0.0258  pu_Lls=0.0413  Rrd=0.009857*10 Ohm  Xlrd=0.04280*10 Ohm  pu_Rrd=0.0145  pu_Llrd=0.0424  Rrd1=0.28 Ohm  Xlrd1=0.82 Ohm  Rrd2=0.28 Ohm  Xlrd2=0.82 Ohm  pu_Rrd1=0.0290  pu_Llrd1=0.0848  pu_Rrd2=0.0290  pu_Llrd2=0.0848  Xm=111.90*10 Ohm  pu_Lm=1.7562  X0=0.4*7 Ohm  pu_L0=0.0413  saturation_option=ee.enum.saturation.exclude  saturation_i=[0, 4, 9, 18, 25, 34, 50, 68, 95, 120] A  saturation_v=[0, 88, 154, 198, 220, 242, 264, 286, 308, 327] V  pu_saturation_i=[0, .176, .396, .792, 1.1, 1.496, 2.2, 2.992, 4.18, 5.28]  pu_saturation_v=[0, .4, .7, .9, 1, 1.1, 1.2, 1.3, 1.4, 1.4864]  connection_option=ee.enum.Connection.delta1  angular_position_specify=off  angular_position_priority=None  angular_position=0 deg  angular_position_nominal_specify=off  angular_position_nominal_value=1  angular_position_nominal_unit=deg  pu_psids_specify=off  pu_psids_priority=None  pu_psids=0  pu_psids_nominal_specify=off  pu_psids_nominal_value=1  pu_psids_nominal_unit=1  pu_psiqs_specify=off  pu_psiqs_priority=None  pu_psiqs=0  pu_psiqs_nominal_specify=off  pu_psiqs_nominal_value=1  pu_psiqs_nominal_unit=1  pu_psi0s_specify=off  pu_psi0s_priority=None  pu_psi0s=0  pu_psi0s_nominal_specify=off  pu_psi0s_nominal_value=1  pu_psi0s_nominal_unit=1  pu_psidr_specify=off  pu_psidr_priority=None  pu_psidr=0  pu_psidr_nominal_specify=off  pu_psidr_nominal_value=1  pu_psidr_nominal_unit=1  pu_psiqr_specify=off  pu_psiqr_priority=None  pu_psiqr=0  pu_psiqr_nominal_specify=off  pu_psiqr_nominal_value=1  pu_psiqr_nominal_unit=1  pu_psidr1_specify=off  pu_psidr1_priority=None  pu_psidr1=0  pu_psidr1_nominal_specify=off  pu_psidr1_nominal_value=1  pu_psidr1_nominal_unit=1  pu_psiqr1_specify=off  pu_psiqr1_priority=None  pu_psiqr1=0  pu_psiqr1_nominal_specify=off  pu_psiqr1_nominal_value=1  pu_psiqr1_nominal_unit=1  pu_psidr2_specify=off  pu_psidr2_priority=None  pu_psidr2=0  pu_psidr2_nominal_specify=off  pu_psidr2_nominal_value=1  pu_psidr2_nominal_unit=1  pu_psiqr2_specify=off  pu_psiqr2_priority=None  pu_psiqr2=0  pu_psiqr2_nominal_specify=off  pu_psiqr2_nominal_value=1  pu_psiqr2_nominal_unit=1  psids_specify=off  psids_priority=None  psids=0 Wb  psids_nominal_specify=off  psids_nominal_value=1  psids_nominal_unit=Wb  psiqs_specify=off  psiqs_priority=None  psiqs=0 Wb  psiqs_nominal_specify=off  psiqs_nominal_value=1  psiqs_nominal_unit=Wb  psi0s_specify=off  psi0s_priority=None  psi0s=0 Wb  psi0s_nominal_specify=off  psi0s_nominal_value=1  psi0s_nominal_unit=Wb  psidr_specify=off  psidr_priority=None  psidr=0 Wb  psidr_nominal_specify=off  psidr_nominal_value=1  psidr_nominal_unit=Wb  psiqr_specify=off  psiqr_priority=None  psiqr=0 Wb  psiqr_nominal_specify=off  psiqr_nominal_value=1  psiqr_nominal_unit=Wb  psidr1_specify=off  psidr1_priority=None  psidr1=0 Wb  psidr1_nominal_specify=off  psidr1_nominal_value=1  psidr1_nominal_unit=Wb  psiqr1_specify=off  psiqr1_priority=None  psiqr1=0 Wb  psiqr1_nominal_specify=off  psiqr1_nominal_value=1  psiqr1_nominal_unit=Wb  psidr2_specify=off  psidr2_priority=None  psidr2=0 Wb  psidr2_nominal_specify=off  psidr2_nominal_value=1  psidr2_nominal_unit=Wb  psiqr2_specify=off  psiqr2_priority=None  psiqr2=0 Wb  psiqr2_nominal_specify=off  psiqr2_nominal_value=1  psiqr2_nominal_unit=Wb  slip_specify=off  slip_priority=None  slip=1  slip_nominal_specify=off  slip_nominal_value=1  slip_nominal_unit=1  real_power_generated_specify=off  real_power_generated_priority=None  real_power_generated=0 W  real_power_generated_nominal_specify=off  real_power_generated_nominal_value=1  real_power_generated_nominal_unit=W  mechanical_power_consumed_specify=off  mechanical_power_consumed_priority=None  mechanical_power_consumed=0 W  mechanical_power_consumed_nominal_specify=off  mechanical_power_consumed_nominal_value=1  mechanical_power_consumed_nominal_unit=W  Tmeas=298.15 K  alpha=3.93e-3 1/K  alpha_cage=4.4e-3 1/K  stator_thermal_mass=100 J/K  rotor_thermal_mass=200 J/K  temperatureA_specify=off  temperatureA_priority=High  temperatureA=25 degC  temperatureA_nominal_specify=off  temperatureA_nominal_value=1  temperatureA_nominal_unit=degC  temperatureB_specify=off  temperatureB_priority=High  temperatureB=25 degC  temperatureB_nominal_specify=off  temperatureB_nominal_value=1  temperatureB_nominal_unit=degC  temperatureC_specify=off  temperatureC_priority=High  temperatureC=25 degC  temperatureC_nominal_specify=off  temperatureC_nominal_value=1  temperatureC_nominal_unit=degC  temperatureR_specify=off  temperatureR_priority=High  temperatureR=25 degC  temperatureR_nominal_specify=off  temperatureR_nominal_value=1  temperatureR_nominal_unit=degC
      settings: InternalSimscapePortConfiguration="{\"Bottom\":[],\"Left\":[{\"id\":\"R\",\"label\":\"R\",\"type\":\"foundation.mechanical.rotational.rotational\"},{\"id\":\"C\",\"label\":\"C\",\"type\":\"foundation.mechanical.rotational.rotational\"}],\"Right\":[{\"id\":\"pu_output\",\"label\":\"pu\",\"type\":\"output\"},{\"id\":\"N1\",\"label\":\"~1\",\"type\":\"foundation.electrical.three_phase\"},{\"id\":\"N2\",\"label\":\"~2\",\"type\":\"foundation.electrical.three_phase\"}],\"Top\":[]}"
  Grounded Neutral (Three-Phase) : ee_lib/Connectors & References/Grounded Neutral (Three-Phase)
  Subsystem : Subsystem
  ~ : PMIOPort  Side=Right
  connections:
  Subsystem/LConn2 -- Asynchronous Machine Squirrel Cage (fundamental)/LConn2
  Subsystem/LConn1 -- Asynchronous Machine Squirrel Cage (fundamental)/LConn1
  Asynchronous Machine Squirrel Cage (fundamental)/RConn2 -- ~/RConn1
  Grounded Neutral (Three-Phase)/LConn1 -- Asynchronous Machine Squirrel Cage (fundamental)/RConn3

== system MicrogridControl/Solar/Solar Plant Integrated ==
  Ir : Inport
  T : Inport  Port=2
  Pref : Inport  Port=3
  Qref : Inport  Port=4
  Mode : Inport  Port=5
  Detailed : Subsystem  VariantControl=Detailed
  Simplified : Subsystem  VariantControl=Simplified
  ~ : PMIOPort  Side=Right
  Meas : Outport

== system MicrogridControl/Solar/Solar Plant Integrated1 ==
  Ir : Inport
  T : Inport  Port=2
  Pref : Inport  Port=3
  Qref : Inport  Port=4
  Mode : Inport  Port=5
  Detailed : Subsystem  VariantControl=Detailed
  Simplified : Subsystem  VariantControl=Simplified
  ~ : PMIOPort  Side=Right
  Meas : Outport

== system MicrogridControl/Solar/Transformer ==
  Detailed : Subsystem  VariantControl=Detailed
  Simplified : Subsystem  VariantControl=Simplified  mask{windingRatio=690/6600}
      mask prompts: windingRatio "Winding ratio"
      mask DialogControl Container4 Prompt: General
  In : PMIOPort  Side=Left
  Out : PMIOPort  Port=2  Side=Right

== system MicrogridControl/Solar/Transformer1 ==
  Detailed : Subsystem  VariantControl=Detailed
  Simplified : Subsystem  VariantControl=Simplified  mask{windingRatio=690/6600}
      mask prompts: windingRatio "Winding ratio"
      mask DialogControl Container4 Prompt: General
  In : PMIOPort  Side=Left
  Out : PMIOPort  Port=2  Side=Right
